simulink model "KITTdyn_speed"  (R2018a)
settings: Solver=FixedStepAuto  StartTime=0.0  FixedStep=0.001  MaxStep=0.01  RelTol=1e-3
values from neighbouring files (symbols this model uses):
  a = 10.44    [mat_creations.m]
  b = 15.83    [mat_creations.m]
  c = 4.954    [mat_creations.m]
  m = 13    [mat_creations.m]
undefined symbols (not defined in the file or in its folder): F_ext
settings Model: Creator=Maarteq  LastModifiedBy=Daan
settings CodeAppCC: StateflowObjectComments=on

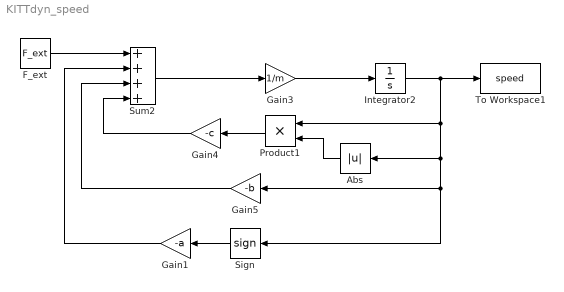
== system KITTdyn_speed ==
  Abs : Abs
  "F_ext " : Constant  Value=F_ext
  Gain1 : Gain  Gain=-a
  Gain3 : Gain  Gain=1/m
  Gain4 : Gain  Gain=-c
  Gain5 : Gain  Gain=-b
  Integrator2 : Integrator
  Product1 : Product
  Sign : Signum
  Sum2 : Sum  Inputs=++++
  To Workspace1 : ToWorkspace  VariableName=speed  SaveFormat=Timeseries  SampleTime=-1
  wires:
  Product1/1 -> Gain4/1
  Gain4/1 -> Sum2/4
  Gain5/1 -> Sum2/3
  Sum2/1 -> Gain3/1
  "F_ext "/1 -> Sum2/1
  Abs/1 -> Product1/2
  Gain3/1 -> Integrator2/1
  Sign/1 -> Gain1/1
  Gain1/1 -> Sum2/2
  Integrator2/1 -> Product1/1, Abs/1, Gain5/1, Sign/1, To Workspace1/1
